simulink subsystem "onboad_env_modelling"  (R2024a)
settings: Solver=VariableStepAuto  StartTime=0.0  StopTime=10.0  RelTol=1e-3
undefined symbols (not defined in the file or in its folder): WMM2020
libraries: matrix_library x1, aerolibtransform2 x1, aerolibutil x1, vrlib x1, aerolibgravity2 x1
settings Model: Creator=joshu  LastModifiedBy=joshu

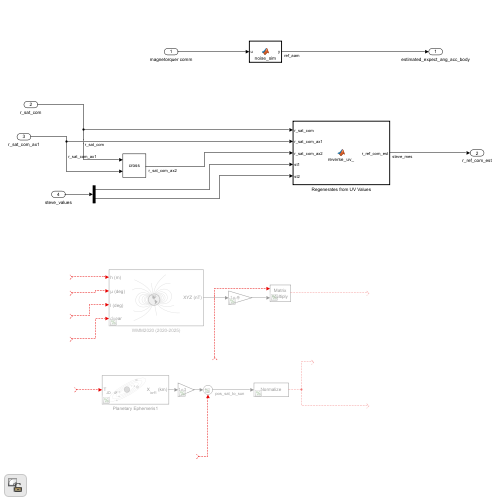
[thumbnail: Simulink's stored preview of the top-level diagram]
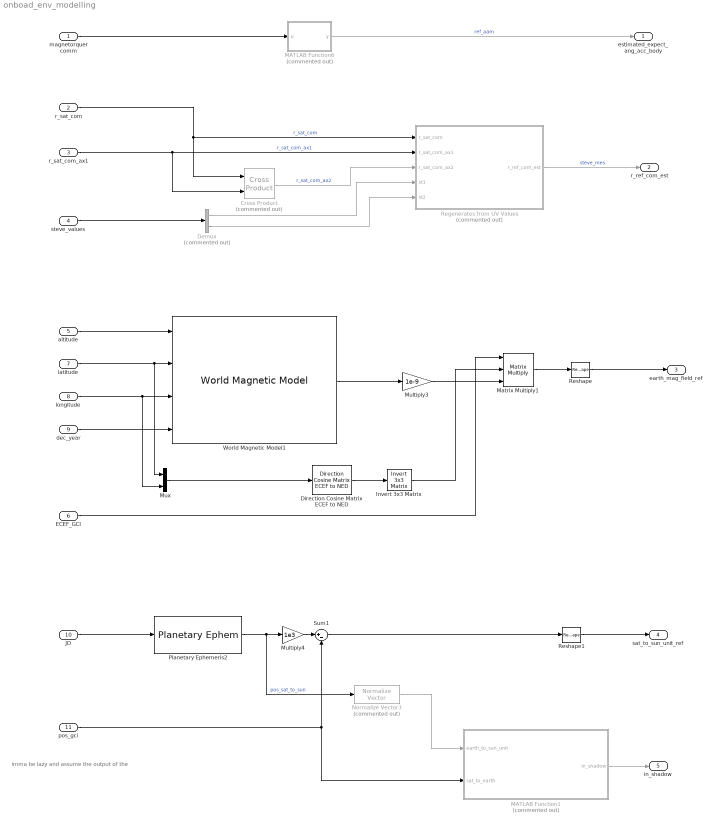
== system onboad_env_modelling ==
  note: imma be lazy and assume the output of the
  magnetorquer comm : Inport
  r_sat_com : Inport  Port=2
  r_sat_com_ax1 : Inport  Port=3
  steve_values : Inport  Port=4
  altitude : Inport  Port=5
  ECEF_GCI : Inport  Port=6
  latitude : Inport  Port=7
  longitude : Inport  Port=8
  dec_year : Inport  Port=9
  JD : Inport  Port=10
  pos_gci : Inport  Port=11
  Cross Product : matrix_library/Cross Product  Commented=on
  Demux : Demux  Commented=on  Outputs=2
  Direction Cosine Matrix ECEF to NED : aerolibtransform2/Direction Cosine Matrix ECEF to NED
  Invert 3x3 Matrix : aerolibutil/Invert  3x3 Matrix
  MATLAB Function1 : MATLAB Function  Commented=on  TreatAsAtomicUnit=on
  MATLAB Function6 : MATLAB Function  Commented=on  TreatAsAtomicUnit=on
  Matrix Multiply1 : Product  Inputs=3  Multiplication=Matrix(*)
  Multiply3 : Gain  Gain=1e-9
  Multiply4 : Gain  Gain=1e3
  Mux : Mux  Inputs=2
  Normalize Vector3 : vrlib/Utilities/Normalize Vector  Commented=on  maxzero=0
  Planetary Ephemeris2 : PlanetaryEphem  target=Sun  outputVelocity=off
  Regenerates from UV Values : MATLAB Function  Commented=on  TreatAsAtomicUnit=on
  Reshape : Reshape  OutputDimensionality=Row vector (2-D)
  Reshape1 : Reshape  OutputDimensionality=Row vector (2-D)
  Sum1 : Sum  Inputs=|+-
  World Magnetic Model1 : aerolibgravity2/World Magnetic Model  model=WMM2020 (2020-2025)  customFile='WMM2020.COF'  units=Metric (MKS)  time_in=on  month=January  day=1  year=2020  action=Warning  h_out=off  dec_out=off  inc_out=off  ti_out=off
  estimated_expect_ang_acc_body : Outport
  r_ref_com_est : Outport  Port=2
  earth_mag_field_ref : Outport  Port=3
  sat_to_sun_unit_ref : Outport  Port=4
  in_shadow : Outport  Port=5
  wires:
  MATLAB Function6/1(y) -> estimated_expect_ang_acc_body/1  "ref_aam"
  magnetorquer comm/1 -> MATLAB Function6/1(u)
  Demux/1 -> Regenerates from UV Values/4(st1)
  Demux/2 -> Regenerates from UV Values/5(st2)
  Regenerates from UV Values/1(r_ref_com_est) -> r_ref_com_est/1  "steve_mes"
  Cross Product/1 -> Regenerates from UV Values/3(r_sat_com_ax2)  "r_sat_com_ax2"
  r_sat_com_ax1/1 -> Cross Product/2, Regenerates from UV Values/2(r_sat_com_ax1)  "r_sat_com_ax1"
  r_sat_com/1 -> Cross Product/1, Regenerates from UV Values/1(r_sat_com)  "r_sat_com"
  steve_values/1 -> Demux/1
  Normalize Vector3/1 -> MATLAB Function1/1(earth_to_sun_unit)
  Mux/1 -> Direction Cosine Matrix ECEF to NED/1
  altitude/1 -> World Magnetic Model1/1
  MATLAB Function1/1(in_shadow) -> in_shadow/1
  Planetary Ephemeris2/1 -> Multiply4/1, Normalize Vector3/1  "pos_sat_to_sun"
  ECEF_GCI/1 -> Matrix Multiply1/1
  latitude/1 -> Mux/1, World Magnetic Model1/2
  Matrix Multiply1/1 -> Reshape/1
  Direction Cosine Matrix ECEF to NED/1 -> Invert 3x3 Matrix/1
  dec_year/1 -> World Magnetic Model1/4
  Sum1/1 -> Reshape1/1
  Multiply3/1 -> Matrix Multiply1/3
  Reshape/1 -> earth_mag_field_ref/1
  JD/1 -> Planetary Ephemeris2/1
  pos_gci/1 -> Sum1/2, MATLAB Function1/2(sat_to_earth)
  Multiply4/1 -> Sum1/1
  longitude/1 -> World Magnetic Model1/3, Mux/2
  World Magnetic Model1/1 -> Multiply3/1
  Invert 3x3 Matrix/1 -> Matrix Multiply1/2
  Reshape1/1 -> sat_to_sun_unit_ref/1

== matlab function onboad_env_modelling/MATLAB Function1 ==
  data: earth_to_sun_unit input; in_shadow output; sat_to_earth input
function in_shadow = is_in_shadow_(earth_to_sun_unit,sat_to_earth)

in_shadow = is_in_shadow(earth_to_sun_unit,sat_to_earth);

== matlab function onboad_env_modelling/MATLAB Function6 ==
  data: u input; y output
function y = noise_sim(u)

y = u;

== matlab function onboad_env_modelling/Regenerates from UV Values ==
  data: r_sat_com input; r_ref_com_est output; r_sat_com_ax1 input; r_sat_com_ax2 input; st1 input; st2 input
function r_ref_com_est = reverse_uv_(r_sat_com,r_sat_com_ax1, ...
                                          r_sat_com_ax2,st1,st2)

r_ref_com_est = reverse_uv(r_sat_com,r_sat_com_ax1,r_sat_com_ax2,st1,st2);
